simulink model "tremolo3"  (R2025b)
settings: Solver=FixedStepDiscrete  StartTime=0.0  StopTime=inf  RelTol=1e-3
undefined symbols (not defined in the file): iPhase_rt, Rate_rt, WaveSel_rt
settings Model: Creator=linogarciamorales  LastModifiedBy=linogarciamorales
settings OptimizationCC: EnhancedBackFolding=on  PassReuseOutputArgsAs=Individual arguments  ZeroExternalMemoryAtStartup=off  ZeroInternalMemoryAtStartup=off  OptimizeBlockOrder=speed  DifferentSizesBufferReuse=on  OptimizationCustomize=off  EfficientTunableParamExpr=on
settings DebuggingCC: ParameterTunabilityLossMsg=error
settings HardwareCC: ProdBitPerPointer=32.0  ProdBitPerSizeT=32.0  ProdBitPerPtrDiffT=32.0  ProdLargestAtomicFloat=None  ProdIntDivRoundTo=Undefined  ProdEndianess=Unspecified  ProdWordSize=32.0  ProdHWDeviceType=Generic->32-bit Embedded Processor
settings SFSimCC: MATLABDynamicMemAlloc=off
settings RTWCC: SystemTargetFile=ert.tlc  GenCodeOnly=on  TemplateMakefile=ert_default_tmf  Description=Embedded Coder
settings CodeAppCC: ForceParamTrailComments=on  IgnoreCustomStorageClasses=off  OperatorAnnotations=on  SimulinkDataObjDesc=on  SFDataObjDesc=on  InsertBlockDesc=on
settings ERTTargetCC: InlinedParameterPlacement=Hierarchical  ERTCustomFileTemplate=example_file_process.tlc  TargetLangStandard=C99 (ISO)  SupportNonInlinedSFcns=on

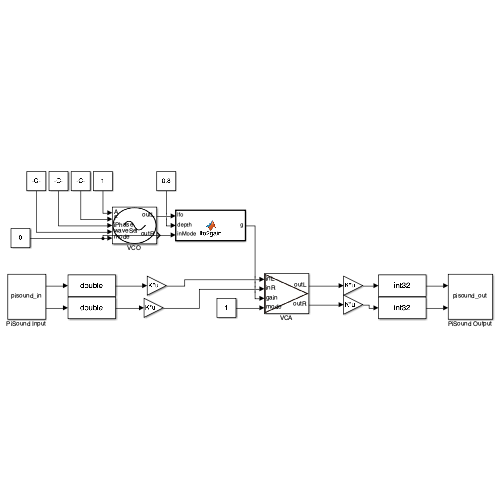
[thumbnail: Simulink's stored preview of the top-level diagram]
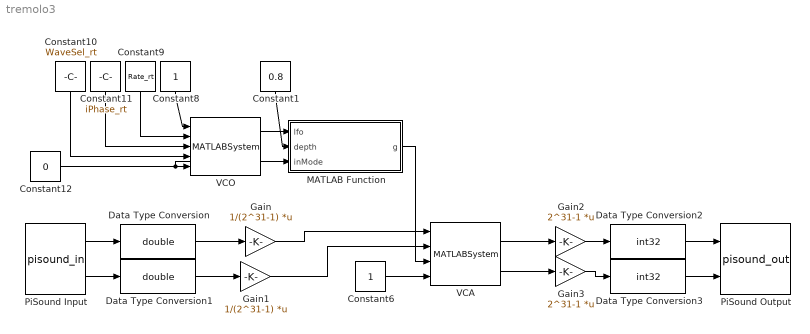
== system tremolo3 ==
  Constant1 : Constant  Value=0.8  OutDataTypeStr=double
  Constant10 : Constant  Value=WaveSel_rt  OutDataTypeStr=uint8
  Constant11 : Constant  Value=iPhase_rt  OutDataTypeStr=double
  Constant12 : Constant  Value=0  OutDataTypeStr=uint8
  Constant6 : Constant  OutDataTypeStr=uint8
  Constant8 : Constant  OutDataTypeStr=double
  Constant9 : Constant  Value=Rate_rt  OutDataTypeStr=double
  Data Type Conversion : DataTypeConversion  OutDataTypeStr=double  SaturateOnIntegerOverflow=off  RndMeth=Floor
  Data Type Conversion1 : DataTypeConversion  OutDataTypeStr=double  SaturateOnIntegerOverflow=off  RndMeth=Floor
  Data Type Conversion2 : DataTypeConversion  OutDataTypeStr=int32  SaturateOnIntegerOverflow=off  RndMeth=Floor
  Data Type Conversion3 : DataTypeConversion  OutDataTypeStr=int32  SaturateOnIntegerOverflow=off  RndMeth=Floor
  Gain : Gain  Gain=1/(2^31-1)  Multiplication=Matrix(K*u)
  Gain1 : Gain  Gain=1/(2^31-1)  Multiplication=Matrix(K*u)
  Gain2 : Gain  Gain=2^31-1  Multiplication=Matrix(K*u)
  Gain3 : Gain  Gain=2^31-1  Multiplication=Matrix(K*u)
  MATLAB Function : MATLAB Function  TreatAsAtomicUnit=on
  PiSound Input : S-Function  FunctionName=pisound_in  Parameters=48000, 128, 0  SFunctionDeploymentMode=off  EnableBusSupport=off
  PiSound Output : S-Function  FunctionName=pisound_out  Parameters=48000, 128, 0  SFunctionDeploymentMode=off  EnableBusSupport=off
  VCA : MATLABSystem  System=vca_sys  N=128  Fs=48000  bypass=uint8(0)  SimulateUsing=Code generation
      mask Type: vca_sys
  VCO : MATLABSystem  System=vco_sys  N=128  Fs=48000  OutMaxL=4096  InFixL=1024  SimulateUsing=Code generation
      mask Type: vco_sys
  wires:
  PiSound Input/1 -> Data Type Conversion/1
  PiSound Input/2 -> Data Type Conversion1/1
  Data Type Conversion/1 -> Gain/1
  Data Type Conversion1/1 -> Gain1/1
  Gain2/1 -> Data Type Conversion2/1
  Gain3/1 -> Data Type Conversion3/1
  Data Type Conversion2/1 -> PiSound Output/1
  Data Type Conversion3/1 -> PiSound Output/2
  Gain/1 -> VCA/1
  VCA/1 -> Gain2/1
  VCA/2 -> Gain3/1
  Gain1/1 -> VCA/2
  Constant6/1 -> VCA/4
  Constant8/1 -> VCO/1
  Constant9/1 -> VCO/2
  Constant10/1 -> VCO/4
  Constant11/1 -> VCO/3
  Constant12/1 -> MATLAB Function/3(inMode), VCO/5
  VCO/1 -> MATLAB Function/1(lfo)
  MATLAB Function/1(g) -> VCA/3
  Constant1/1 -> MATLAB Function/2(depth)

== matlab function tremolo3/MATLAB Function ==
  data: lfo input; g output; depth input; inMode input
function g = lfo2gain(lfo, depth, inMode)
%#codegen
% lfo    : Nx1 (double)  (en tu caso N=128)
% depth  : escalar 0..1
% inMode : 0=bipolar [-1,1], 1=unipolar [0,1]
%
% salida g: Nx1 en [1-depth, 1]

% clamp depth
if depth < 0, depth = 0; end
if depth > 1, depth = 1; end

N = 128;                 % <-- fijo (tu frame)
g = zeros(N,1);

m = (inMode ~= 0);       % fuerza 0/1

if m
    % unipolar [0,1] -> [1-depth, 1]
    for i = 1:N
        x = lfo(i);
        if x < 0, x = 0; end
        if x > 1, x = 1; end
        g(i) = (1 - depth) + depth*x;
    end
else
    % bipolar [-1,1] -> [1-depth, 1]
    for i = 1:N
        x = lfo(i);
        if x < -1, x = -1; end
        if x >  1, x =  1; end
        g(i) = (1 - 0.5*depth) + (0.5*depth)*x;
    end
end
end
